simulink library "CommandFilter"  (R2013b)
settings: Solver=ode45  StartTime=0.0  StopTime=10.0  RelTol=1e-3
settings Model: Creator=Nam  LastModifiedBy=Nam

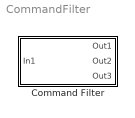
== system CommandFilter ==
  Command Filter : Subsystem  mask{Integrator1_init=0, omega_n=2*pi*1, zeta=.5}
      mask init:
      | zeta > 0
      | zeta <= 1
      mask DialogControl Control3 Prompt: Initial value Integrator1
      mask DialogControl Control5 Prompt: omega_n
      mask DialogControl Control4 Prompt: zeta

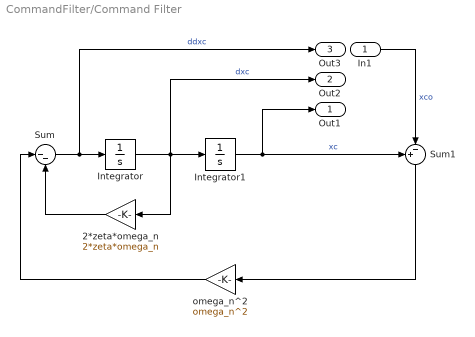
== system CommandFilter/Command Filter ==
  In1 : Inport
  2*zeta*omega_n : Gain  Gain=2*zeta*omega_n
  Integrator : Integrator
  Integrator1 : Integrator  InitialCondition=Integrator1_init
  Sum : Sum  Inputs=|--
  Sum1 : Sum  Inputs=+-|
  omega_n^2 : Gain  Gain=omega_n^2
  Out1 : Outport
  Out2 : Outport  Port=2
  Out3 : Outport  Port=3
  wires:
  Sum/1 -> Out3/1, Integrator/1  "ddxc"
  In1/1 -> Sum1/2  "xco"
  2*zeta*omega_n/1 -> Sum/2
  Integrator/1 -> Out2/1, 2*zeta*omega_n/1, Integrator1/1  "dxc"
  omega_n^2/1 -> Sum/1
  Sum1/1 -> omega_n^2/1
  Integrator1/1 -> Out1/1, Sum1/1  "xc"
